simulink library "engine_AMT180_lib"  (Simulink 7.2)
settings: Solver=ode45  SolverMode=SingleTasking  StartTime=0.0  StopTime=10.0  RelTol=1e-3
libraries: simulink_need_slupdate x4, simulink x1
settings Model: Creator=amurch  LastModifiedBy=amurch

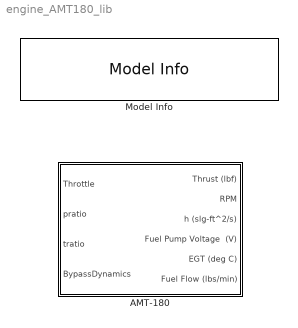
== system engine_AMT180_lib ==
  AMT-180 : Subsystem
      mask init:
      | % GTM engine, steady-state bench data.
      | %"Miniature Gas Turbine Engine Evaluation Study"
      | % Greg Howland, Internal Report, July 29,2002.
      | 
      | % 1st-Run data set, used in GTMsim
      | %Throttle_bpt = [8,15,22,31,36,39,46,53.5,61,77,92,100];
      | %Thrust_tbl = [1.86,2.66,3.69,5.14,6.19,6.79,8.38,9.91,11.43,14.42,16.71,17.78];
      | %RPM_tbl    = 1000*[60.9, 71.4, 82.6, 95.9, 102.9, 107.1, 116.2, 123.9, 130.2, 142.1, 149.1, 151.2];
      | 
      | % 2nd-Run data set
      | Throttle_bpt = [0.00 6.00 12.00 19.00 24.00 30.00 33.00 37.00 42.00 48.00 54.50 60.00 66.00 72.00 84.00 100.00];%percent
      | Thrust_tbl   = [1.20 1.79 2.35 3.16 3.98 5.05 5.70 6.49 7.70 9.00 9.68 10.65 11.72 12.81 15.44 17.89];%lbs
      | RPM_tbl      = 1000*[49.00 58.80 66.50 77.00 85.40 94.50 99.40 105.70 112.70 119.70 122.50 127.40 131.60 135.80 144.90 151.90 ]; %rot/min
      | FuelFlow_tbl = 1/12*[2.74 3.18 3.62 4.16 4.60 5.31 5.71 6.25 6.99 7.54 7.77 8.38 8.82 9.19 10.41 12.23]; %lbs/min
      | 
      | % 2nd order time constant.
      | rpm_bpt=[ 0 61000 100000  160000];
      | wn_tbl     =2*pi*[.2  .2   .4     .7];
      | zeta_tbl   =[.9   .75    .65     .6];
      | 
      | %Tau    = 1.02; % SWAG - taken from AMT-280 data  at 75% throttle
      | 
      | % Equvalent Shaft parameters for engine
      | shaft_dia = 0.75/12.0;       % diameter of rotating turbine in feet 
      | shaft_len = 6.25/12.0;       % length of rotating turbine in feet   
      | density   = 15.2;            % mass density of steel in slugs/ft^3 
      | 
      | fuelpump_table = [ 0.90 1.0 6.4]; %volts, table of fuel pump voltages  - not accurate at the moment 2-4-08
      | fuelflow_table = [0.00 0.1762 1.34044]; %lbs/min,   fuel flow rates corresponding to pump voltages (pumpv_table)
  Model Info : simulink/Model-Wide Utilities/Model Info  SystemSampleTime=-1  InitialBlockCM=None  BlockCM=None  Frame=on  DisplayStringWithTags=|  HorizontalTextAlignment=Center  LeftAlignmentValue=0.5  SourceBlockDiagram=engine_AMT180_lib  TagMaxNumber=20
      | AMT-180 Engine Library
      | 
      | Model Version: %<ModelVersion>
      | Last modifed by %<LastModifiedBy> on %<LastModificationDate>

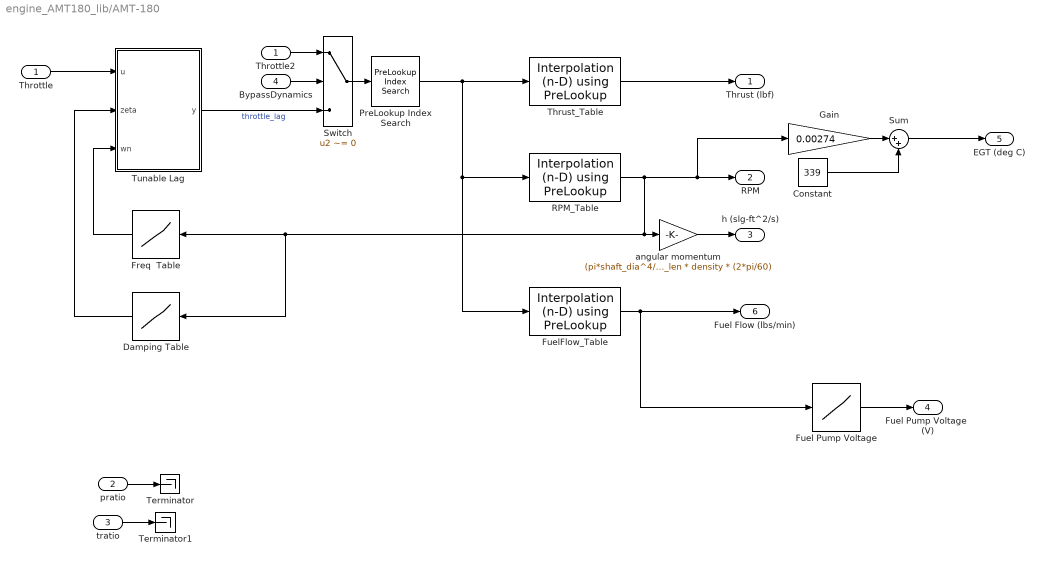
== system engine_AMT180_lib/AMT-180 ==
  Throttle : Inport  OutDataType=sfix(16)  OutScaling=2^0
  pratio : Inport  Port=2  OutDataType=sfix(16)  OutScaling=2^0
  tratio : Inport  Port=3  OutDataType=sfix(16)  OutScaling=2^0
  BypassDynamics : Inport  Port=4  OutDataType=sfix(16)  OutScaling=2^0
  Constant : Constant  Value=339  OutDataType=sfix(16)  OutScaling=2^0
  Damping Table : Lookup  Orientation=left  InputValues=rpm_bpt  Table=zeta_tbl  LookUpMeth=Interpolation-Use End Values  OutDataType=sfix(16)  OutScaling=2^0
  Freq  Table : Lookup  Orientation=left  InputValues=rpm_bpt  Table=wn_tbl  LookUpMeth=Interpolation-Use End Values  OutDataType=sfix(16)  OutScaling=2^0
  Fuel Pump Voltage : Lookup  InputValues=fuelflow_table  Table=fuelpump_table  LookUpMeth=Interpolation-Use End Values  OutDataType=sfix(16)  OutScaling=2^0
  FuelFlow_Table : simulink_need_slupdate/Interpolation (n-D) using PreLookup  numDimsPopupSelect=1  explicitNumDims=2  table=FuelFlow_tbl  interpMethod=Linear  extrapMethod=Linear  rangeErrorMode=None  NumSelectionDims=0
  Gain : Gain  Gain=0.00274  ParameterDataType=sfix(16)  ParameterScaling=2^0  OutDataType=sfix(16)  OutScaling=2^0
  PreLookup Index Search : simulink_need_slupdate/PreLookup Index Search  bpData=Throttle_bpt  searchMode=Binary Search  cacheBpFlag=off  outputFlag=off  IndexDataType=uint32  extrapMode=Clip to Range  rangeErrorMode=None
  RPM_Table : simulink_need_slupdate/Interpolation (n-D) using PreLookup  numDimsPopupSelect=1  explicitNumDims=2  table=RPM_tbl  interpMethod=Linear  extrapMethod=Linear  rangeErrorMode=None  NumSelectionDims=0
  Sum : Sum  Inputs=|++  OutDataType=sfix(16)  OutScaling=2^0
  Switch : Switch  Criteria=u2 ~= 0
  Terminator : Terminator
  Terminator1 : Terminator
  Throttle2 : InportShadow  Port=1  OutDataType=sfix(16)  OutScaling=2^0  LatchByCopyingInsideSignal=off
  Thrust_Table : simulink_need_slupdate/Interpolation (n-D) using PreLookup  numDimsPopupSelect=1  explicitNumDims=2  table=Thrust_tbl  interpMethod=Linear  extrapMethod=Linear  rangeErrorMode=None  NumSelectionDims=0
  Tunable Lag : Subsystem
      mask Description:
      | Implements tunable 2nd order all-pole filter:
      | 
      |              Wn^2
      |     -------------------
      |    s^2 + 2*zeta*Wns + Wn^2
  angular momentum : Gain  Gain=(pi*shaft_dia^4/32) * shaft_len * density * (2*pi/60)  ParameterDataType=sfix(16)  ParameterScaling=2^0  OutDataType=sfix(16)  OutScaling=2^0
  Thrust (lbf) : Outport  OutDataType=sfix(16)  OutScaling=2^0
  RPM : Outport  Port=2  OutDataType=sfix(16)  OutScaling=2^0
  h (slg-ft^2/s) : Outport  Port=3  OutDataType=sfix(16)  OutScaling=2^0
  Fuel Pump Voltage  (V) : Outport  Port=4  OutDataType=sfix(16)  OutScaling=2^0
  EGT (deg C) : Outport  Port=5  OutDataType=sfix(16)  OutScaling=2^0
  Fuel Flow (lbs/min) : Outport  Port=6  OutDataType=sfix(16)  OutScaling=2^0
  wires:
  RPM_Table/1 -> angular momentum/1, Freq  Table/1, Damping Table/1, RPM/1, Gain/1
  angular momentum/1 -> h (slg-ft^2/s)/1
  Thrust_Table/1 -> Thrust (lbf)/1
  PreLookup Index Search/1 -> Thrust_Table/1, RPM_Table/1, FuelFlow_Table/1
  FuelFlow_Table/1 -> Fuel Flow (lbs/min)/1, Fuel Pump Voltage/1
  Throttle/1 -> Tunable Lag/1(u)
  Freq  Table/1 -> Tunable Lag/3(wn)
  Damping Table/1 -> Tunable Lag/2(zeta)
  pratio/1 -> Terminator/1
  tratio/1 -> Terminator1/1
  Fuel Pump Voltage/1 -> Fuel Pump Voltage  (V)/1
  Sum/1 -> EGT (deg C)/1
  Constant/1 -> Sum/2
  Gain/1 -> Sum/1
  BypassDynamics/1 -> Switch/2
  Throttle2/1 -> Switch/1
  Tunable Lag/1(y) -> Switch/3  "throttle_lag"
  Switch/1 -> PreLookup Index Search/1

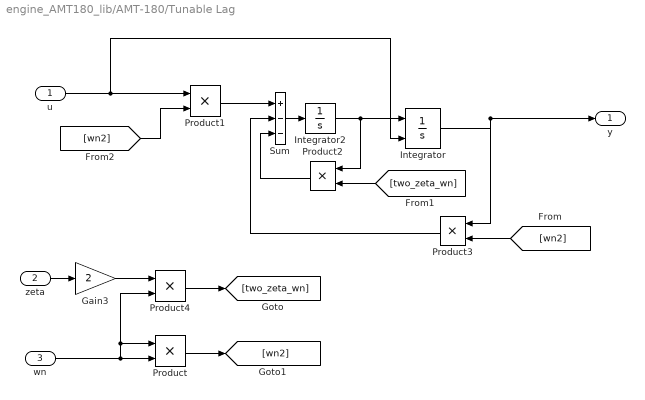
== system engine_AMT180_lib/AMT-180/Tunable Lag ==
  u : Inport  OutDataType=sfix(16)  OutScaling=2^0
  zeta : Inport  Port=2  OutDataType=sfix(16)  OutScaling=2^0
  wn : Inport  Port=3  OutDataType=sfix(16)  OutScaling=2^0
  Gain3 : Gain  Gain=2  ParameterDataType=sfix(16)  ParameterScaling=2^0  OutDataType=sfix(16)  OutScaling=2^0
  Integrator : Integrator  InitialConditionSource=external
  Integrator2 : Integrator
  Product : Product  OutDataType=sfix(16)  OutScaling=2^0  RndMeth=Zero
  Product1 : Product  OutDataType=sfix(16)  OutScaling=2^0  RndMeth=Zero
  Product2 : Product  Orientation=left  OutDataType=sfix(16)  OutScaling=2^0  RndMeth=Zero
  Product3 : Product  Orientation=left  OutDataType=sfix(16)  OutScaling=2^0  RndMeth=Zero
  Product4 : Product  OutDataType=sfix(16)  OutScaling=2^0  RndMeth=Zero
  Sum : Sum  Inputs=+--  OutDataType=sfix(16)  OutScaling=2^0
  y : Outport  OutDataType=sfix(16)  OutScaling=2^0
  wires:
  [wn2] -> Product1/2
  Product/1 -> [wn2]
  Product4/1 -> [two_zeta_wn]
  Gain3/1 -> Product4/1
  zeta/1 -> Gain3/1
  wn/1 -> Product4/2, Product/1, Product/2
  [two_zeta_wn] -> Product2/2
  [wn2] -> Product3/2
  Product2/1 -> Sum/3
  Product3/1 -> Sum/2
  u/1 -> Product1/1, Integrator/2
  Product1/1 -> Sum/1
  Integrator2/1 -> Product2/1, Integrator/1
  Sum/1 -> Integrator2/1
  Integrator/1 -> Product3/1, y/1
